simulink model "My"  (R2017a)
settings: Solver=VariableStepAuto  StartTime=0.0  StopTime=10  RelTol=1e-3
libraries: dspsrcs4 x1
settings Model: Creator=Student  LastModifiedBy=root

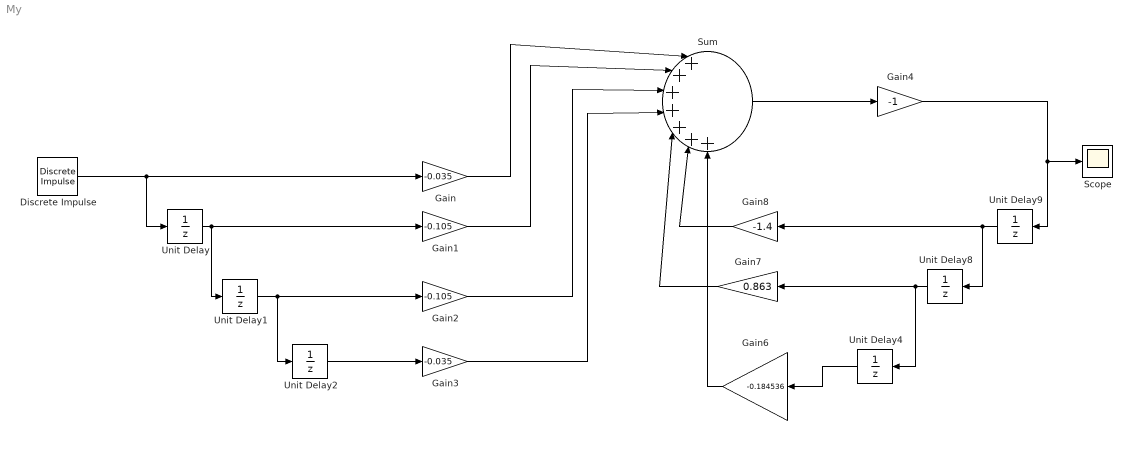
== system My ==
  Discrete Impulse : dspsrcs4/Discrete  Impulse  Delay=0  SampleTime=1  FrameSample=1  OutputFrames=off  dataType=double  isSigned=on  wordLen=16  udDataType=sfix(16)  fracBitsMode=Best precision  numFracBits=15  OutDataTypeStr=double  LastOutDataTypeStr=double
  Gain : Gain  Gain=-0.035
  Gain1 : Gain  Gain=-0.105
  Gain2 : Gain  Gain=-0.105
  Gain3 : Gain  Gain=-0.035
  Gain4 : Gain  Gain=-1
  Gain6 : Gain  Gain=-0.184536
  Gain7 : Gain  Gain=0.863
  Gain8 : Gain  Gain=-1.4
  Scope : Scope
  Sum : Sum  Inputs=|+++++++
  Unit Delay{,1..2,4,8..9} (6 alike) : UnitDelay  SampleTime=-1
  wires:
  Discrete Impulse/1 -> Unit Delay/1, Gain/1
  Unit Delay/1 -> Unit Delay1/1, Gain1/1
  Unit Delay1/1 -> Unit Delay2/1, Gain2/1
  Unit Delay2/1 -> Gain3/1
  Gain/1 -> Sum/1
  Gain1/1 -> Sum/2
  Gain2/1 -> Sum/3
  Gain3/1 -> Sum/4
  Unit Delay4/1 -> Gain6/1
  Gain6/1 -> Sum/7
  Unit Delay8/1 -> Gain7/1, Unit Delay4/1
  Unit Delay9/1 -> Gain8/1, Unit Delay8/1
  Sum/1 -> Gain4/1
  Gain7/1 -> Sum/5
  Gain8/1 -> Sum/6
  Gain4/1 -> Unit Delay9/1, Scope/1
